simulink subsystem "Pupil_Diameter_Model"  (R2020a)
settings: Solver=VariableStepAuto  StartTime=0.0  StopTime=10.0  RelTol=1e-3
libraries: dspstat3 x1
settings Model: Creator=LAB-OREN3  LastModifiedBy=LAB-OREN3

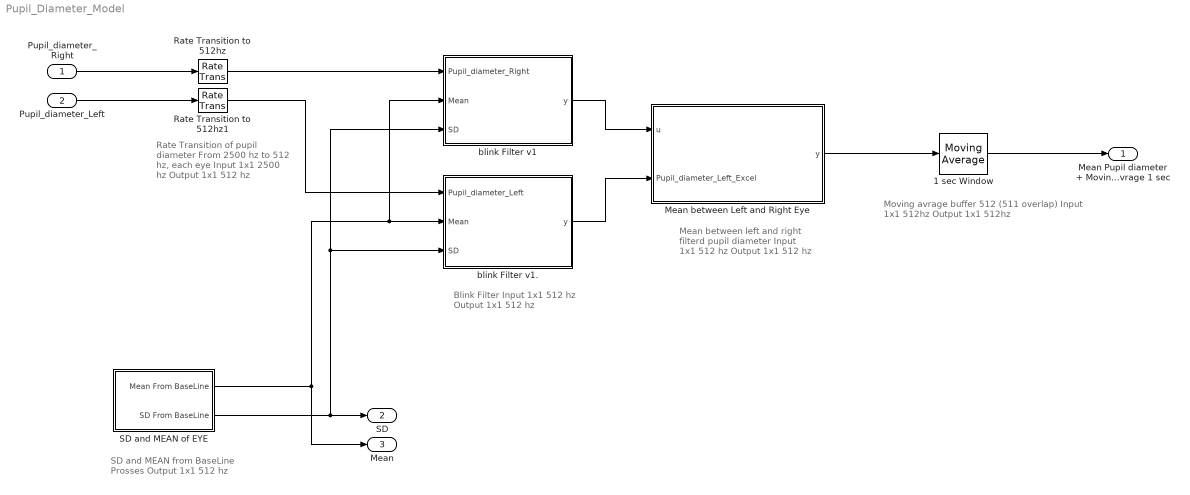
== system Pupil_Diameter_Model ==
  note: Rate Transition of pupil diameter From 2500 hz to 512 hz, each eye
      |
      | Input 1x1 2500 hz
      | Output 1x1 512 hz
  note: Mean between left and right filterd pupil diameter
      |
      | Input 1x1 512 hz
      | Output 1x1 512 hz
  note: Moving avrage buffer 512 (511 overlap)
      |
      | Input 1x1 512hz
      | Output 1x1 512hz
  note: Blink Filter
      |
      | Input 1x1 512 hz
      | Output 1x1 512 hz
  note: SD and MEAN from BaseLine Prosses
      |
      | Output 1x1 512 hz
  Pupil_diameter_Right : Inport
  Pupil_diameter_Left : Inport  Port=2
  1 sec Window : dspstat3/Moving Average  Method=Sliding window  ForgettingFactorPort=off  SpecifyWindowLength=on  WindowLength=512  ForgettingFactor=0.9  SimulateUsing=Code generation
  Mean between Left and Right Eye : MATLAB Function  TreatAsAtomicUnit=on
  Rate Transition to 512hz : RateTransition  Deterministic=off  OutPortSampleTime=0.001953125
  Rate Transition to 512hz1 : RateTransition  Deterministic=off  OutPortSampleTime=0.001953125
  SD and MEAN of EYE : Subsystem
  blink Filter v1 : MATLAB Function  TreatAsAtomicUnit=on
  blink Filter v1. : MATLAB Function  TreatAsAtomicUnit=on
  Mean Pupil diameter + Moving avrage 1 sec : Outport
  SD : Outport  Port=2
  Mean : Outport  Port=3
  wires:
  blink Filter v1/1(y) -> Mean between Left and Right Eye/1(u)
  Mean between Left and Right Eye/1(y) -> 1 sec Window/1
  blink Filter v1./1(y) -> Mean between Left and Right Eye/2(Pupil_diameter_Left_Excel)
  1 sec Window/1 -> Mean Pupil diameter + Moving avrage 1 sec/1
  Pupil_diameter_Left/1 -> Rate Transition to 512hz1/1
  Pupil_diameter_Right/1 -> Rate Transition to 512hz/1
  SD and MEAN of EYE/2(SD From BaseLine) -> SD/1, blink Filter v1/3(SD), blink Filter v1./3(SD)
  SD and MEAN of EYE/1(Mean From BaseLine) -> Mean/1, blink Filter v1/2(Mean), blink Filter v1./2(Mean)
  Rate Transition to 512hz/1 -> blink Filter v1/1(Pupil_diameter_Right)
  Rate Transition to 512hz1/1 -> blink Filter v1./1(Pupil_diameter_Left)

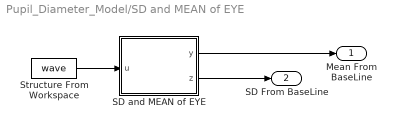
== system Pupil_Diameter_Model/SD and MEAN of EYE ==
  SD and MEAN of EYE : MATLAB Function  TreatAsAtomicUnit=on
  Structure From Workspace : FromWorkspace  VariableName=wave
  Mean From BaseLine : Outport
  SD From BaseLine : Outport  Port=2
  wires:
  SD and MEAN of EYE/1(y) -> Mean From BaseLine/1
  Structure From Workspace/1 -> SD and MEAN of EYE/1(u)
  SD and MEAN of EYE/2(z) -> SD From BaseLine/1

== matlab function Pupil_Diameter_Model/blink Filter v1 ==
  data: Pupil_diameter_Right input; y output; Mean input; SD input
function y = fcn(Pupil_diameter_Right, Mean, SD)
    
  if Pupil_diameter_Right < 2.0 
      y = Mean-(2*SD);
  elseif Pupil_diameter_Right > 8.0
      y = Mean+(2*SD);
  else
      y = Pupil_diameter_Right;
  end
end

== matlab function Pupil_Diameter_Model/blink Filter v1. ==
  data: Pupil_diameter_Left input; y output; Mean input; SD input
function y = fcn(Pupil_diameter_Left, Mean, SD)
    
  if Pupil_diameter_Left < 2.0 
      y = Mean-(2*SD);
  elseif Pupil_diameter_Left > 8.0
      y = Mean+(2*SD);
  else
      y = Pupil_diameter_Left;
  end
end

== matlab function Pupil_Diameter_Model/Mean between Left and Right Eye ==
  data: u input; y output; Pupil_diameter_Left_Excel input
function y = fcn(u, Pupil_diameter_Left_Excel)
 
    
y = (u+Pupil_diameter_Left_Excel)/2;

== matlab function Pupil_Diameter_Model/SD and MEAN of EYE/SD and MEAN of EYE ==
  data: u input; y output; z output
function [y,z]  = func(u)



y = u(1,1);
z = u(2,1);
